simulink model "VanDeVusseMIMO"  (R2017a)
settings: Solver=VariableStepAuto  StartTime=0.0  StopTime=0.1  RelTol=1e-3
values from neighbouring files (symbols this model uses):
  du = 5    [mainVV.m]
settings Model: Creator=Sergio  LastModifiedBy=Sergio

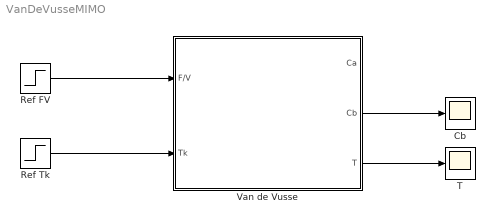
== system VanDeVusseMIMO ==
  Cb : Scope
  Ref FV : Step  Time=0  Before=72  After=72+du  SampleTime=0.005
  Ref Tk : Step  Time=1.5  Before=128.95  After=128.95  SampleTime=0.005
  T : Scope
  Van de Vusse : Subsystem
      mask Display: image('C:\Users\Sergio\Dropbox\UFRJ\DINÂMICA E CONTROLE DE PROCESSOS\Trabalho3\Codigos\VanVUsse.png');
  wires:
  Van de Vusse/2(Cb) -> Cb/1
  Van de Vusse/3(T) -> T/1
  Ref Tk/1 -> Van de Vusse/2(Tk)
  Ref FV/1 -> Van de Vusse/1(F/V)

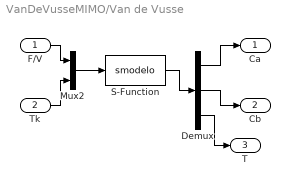
== system VanDeVusseMIMO/Van de Vusse ==
  F/V : Inport
  Tk : Inport  Port=2
  Demux : Demux  Outputs=3
  Mux2 : Mux  Inputs=2
  S-Function : S-Function  FunctionName=smodelo  Parameters="1.287e12,1.287e12,9.043e9, -9758.3, -9758.3, -8560.0, -4.2, 11.0, 41.85, 0.9342, 3.01, 4032.0, 0.215, 5.1, 130.0, 10, 2.4499,    1.1033,  136.7606"  SFunctionDeploymentMode=off  EnableBusSupport=off
  Ca : Outport
  Cb : Outport  Port=2
  T : Outport  Port=3
  wires:
  Demux/3 -> T/1
  F/V/1 -> Mux2/1
  Demux/2 -> Cb/1
  Tk/1 -> Mux2/2
  Demux/1 -> Ca/1
  S-Function/1 -> Demux/1
  Mux2/1 -> S-Function/1
